simulink model "Force_control_compliance"  (R2020b)
settings: Solver=VariableStepAuto  StartTime=0.0  StopTime=10.0  RelTol=1e-3
settings Model: Creator=Anna Rothweil  LastModifiedBy=Anna Rothweil
settings DebuggingCC: UnderSpecifiedDimensionMsg=warning
settings SFSimCC: CustomCodeUndefinedFunction=UseInterfaceOnly

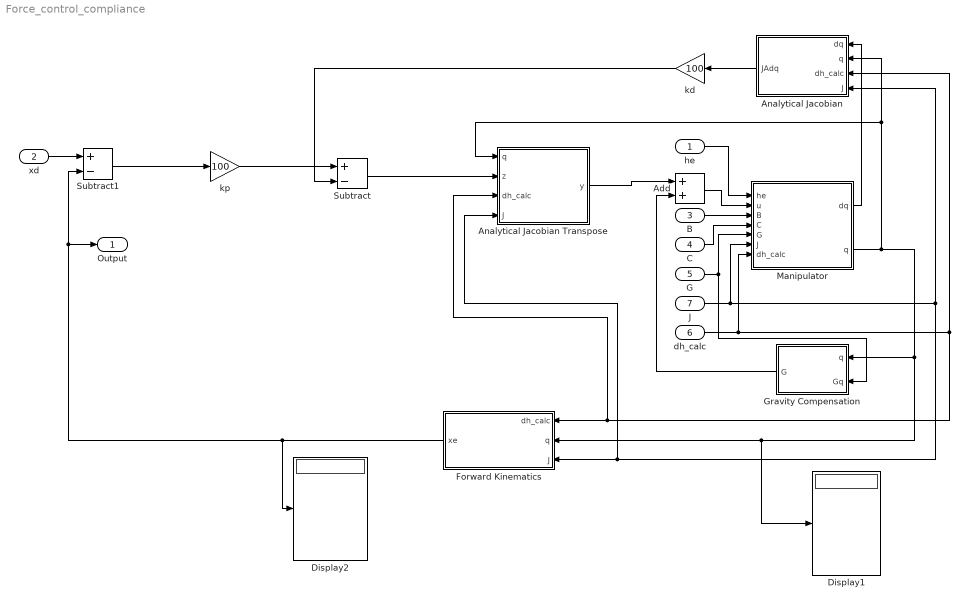
== system Force_control_compliance ==
  he : Inport
  xd : Inport  Port=2
  B : Inport  Port=3
  C : Inport  Port=4
  G : Inport  Port=5
  dh_calc : Inport  Port=6  PortDimensions=12
  J : Inport  Port=7
  Add : Sum
  Analytical Jacobian : MATLAB Function  TreatAsAtomicUnit=on
  "Analytical Jacobian Transpose " : MATLAB Function  TreatAsAtomicUnit=on
  Display1 : Display
  Display2 : Display
  "Forward Kinematics " : MATLAB Function  TreatAsAtomicUnit=on
  "Gravity Compensation " : MATLAB Function  TreatAsAtomicUnit=on
  Manipulator : Subsystem
  Subtract : Sum  Inputs=+-
  Subtract1 : Sum  Inputs=+-
  kd : Gain  Gain=100
  "kp " : Gain  Gain=100
  Output : Outport
  wires:
  Subtract1/1 -> "kp "/1
  "Gravity Compensation "/1(G) -> Add/2
  Subtract/1 -> "Analytical Jacobian Transpose "/2(z)
  "Analytical Jacobian Transpose "/1(y) -> Add/1
  kd/1 -> Subtract/2
  "kp "/1 -> Subtract/1
  xd/1 -> Subtract1/1
  dh_calc/1 -> Manipulator/7(dh_calc), "Analytical Jacobian Transpose "/3(dh_calc), "Forward Kinematics "/1(dh_calc), Analytical Jacobian/3(dh_calc)
  Manipulator/1(dq) -> Analytical Jacobian/1(dq)
  Manipulator/2("q ") -> "Analytical Jacobian Transpose "/1(q), Analytical Jacobian/2(q), Display1/1, "Forward Kinematics "/2(q), "Gravity Compensation "/1(q)
  Add/1 -> Manipulator/2(u)
  he/1 -> Manipulator/1(he)
  "Forward Kinematics "/1(xe) -> Output/1, Subtract1/2, Display2/1
  B/1 -> Manipulator/3(B)
  C/1 -> Manipulator/4(C)
  G/1 -> "Gravity Compensation "/2(Gq), Manipulator/5(G)
  Analytical Jacobian/1(JAdq) -> kd/1
  J/1 -> Manipulator/6(J), "Analytical Jacobian Transpose "/4(J), "Forward Kinematics "/3(J), Analytical Jacobian/4(J)

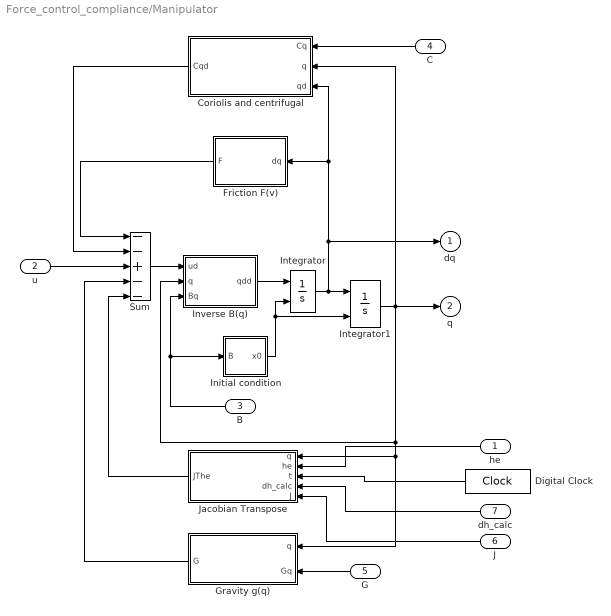
== system Force_control_compliance/Manipulator ==
  he : Inport
  u : Inport  Port=2
  B : Inport  Port=3
  C : Inport  Port=4
  G : Inport  Port=5
  J : Inport  Port=6
  dh_calc : Inport  Port=7
  Coriolis and centrifugal : MATLAB Function  TreatAsAtomicUnit=on
  Digital Clock : DigitalClock  SampleTime=0.001
  Friction F(v) : MATLAB Function  TreatAsAtomicUnit=on
  Gravity g(q) : MATLAB Function  TreatAsAtomicUnit=on
  Initial condition : MATLAB Function  TreatAsAtomicUnit=on
  Integrator : Integrator  InitialConditionSource=external  InitialCondition=[0 0 0 0 0 0]  ZeroCross=off
  Integrator1 : Integrator  InitialConditionSource=external  InitialCondition=[0 0 0 0 0 0]  ZeroCross=off
  Inverse B(q) : MATLAB Function  TreatAsAtomicUnit=on
  Jacobian Transpose : MATLAB Function  TreatAsAtomicUnit=on
  Sum : Sum  Inputs=--+--  InputSameDT=on  SaturateOnIntegerOverflow=on  OutDataTypeStr=Inherit: Same as first input
  dq : Outport  InitialOutput=0
  "q " : Outport  Port=2  InitialOutput=0
  wires:
  Inverse B(q)/1(qdd) -> Integrator/1
  Integrator/1 -> dq/1, Coriolis and centrifugal/3(qd), Friction F(v)/1(dq), Integrator1/1
  Coriolis and centrifugal/1(Cqd) -> Sum/2
  Friction F(v)/1(F) -> Sum/1
  u/1 -> Sum/3
  Integrator1/1 -> Coriolis and centrifugal/2(q), "q "/1, Inverse B(q)/2(q), Gravity g(q)/1(q), Jacobian Transpose/1(q)
  Gravity g(q)/1(G) -> Sum/4
  Jacobian Transpose/1(JThe) -> Sum/5
  he/1 -> Jacobian Transpose/2(he)
  Sum/1 -> Inverse B(q)/1(ud)
  Digital Clock/1 -> Jacobian Transpose/3(t)
  C/1 -> Coriolis and centrifugal/1(Cq)
  B/1 -> Inverse B(q)/3(Bq), Initial condition/1(B)
  G/1 -> Gravity g(q)/2(Gq)
  J/1 -> Jacobian Transpose/5(J)
  dh_calc/1 -> Jacobian Transpose/4(dh_calc)
  Initial condition/1(x0) -> Integrator1/2, Integrator/2

== matlab function Force_control_compliance/Manipulator/Coriolis and centrifugal ==
  data: Cq input; q input; Cqd output; qd input
function Cqd = fcn(Cq, q, qd)
coder.extrinsic('CFinder');
n=size(q, 1);
C = zeros(n,n);
C = CFinder(Cq, q, qd);
Cqd=zeros(n,1);
Cqd=C*qd;

== matlab function Force_control_compliance/Analytical Jacobian Transpose  ==
  data: q input; z input; y output; dh_calc input; J input
function y = fcn(q, z, dh_calc, J)
%dh_calc: the 4*N x 1 vector of symbolic dh parameters (numbers)
%convert dh_calc to matrix form of size Nx4
n=size(q,1);
dh_calc2 = zeros(n,4);
w=1;
for j=1:4
    for i=1:n
        dh_calc2(i,j) = dh_calc(w);
        w=w+1;
    end
end

%z must be 6x1
coder.extrinsic('JAFinder');
JA=zeros(6,n);
JA = JAFinder(dh_calc2, q, J);
y=zeros(n,1);
y=JA.'*z;

== matlab function Force_control_compliance/Forward Kinematics  ==
  data: dh_calc input; q input; xe output; J input
function xe = fcn(dh_calc, q, J)
%dh_calc: the 4*N x 1 vector of symbolic dh parameters (numbers)
%convert dh_calc to matrix form of size Nx4
n=[size(dh_calc,1)]/4;
dh_calc2 = zeros(n,4);
w=1;
for j=1:4
    for i=1:n
        dh_calc2(i,j) = dh_calc(w);
        w=w+1;
    end
end

%q: Nx1 matrix of joint parameters
%T: 4x4 homogeneous transformation matrix

%I think this code is not working because Arm is symbolic
%let's evaluate Arm first before using it with fkine
coder.extrinsic('ArmFinder');
xe=zeros(6,1);
xe = ArmFinder(dh_calc2, q, J);

% s=size(xe,1)
% if s==6
%     xe=xe;
% else
%     xe=zeros(6,1)
%     fprintf('xe is zeros - FWD KIN error')
end

== matlab function Force_control_compliance/Manipulator/Gravity g(q) ==
  data: q input; G output; Gq input
function G = fcn(q, Gq)
coder.extrinsic('GFinder');
n=size(q, 1);
G = zeros(n,1);
G = GFinder(Gq, q);

== matlab function Force_control_compliance/Analytical Jacobian ==
  data: dq input; JAdq output; q input; dh_calc input; J input
function JAdq = fcn(dq, q, dh_calc, J)
%dh_calc: the 4*N x 1 vector of symbolic dh parameters (numbers)
%convert dh_calc to matrix form of size Nx4
n=size(q,1);
dh_calc2 = zeros(n,4);
w=1;
for j=1:4
    for i=1:n
        dh_calc2(i,j) = dh_calc(w);
        w=w+1;
    end
end

coder.extrinsic('JAFinder');
JA=zeros(6,n);
JA = JAFinder(dh_calc2, q, J);
JAdq=zeros(6,1);
JAdq=JA*dq;

== matlab function Force_control_compliance/Gravity Compensation  ==
  data: q input; Gq input; G output
function G = fcn(q, Gq)
n=size(q,1);
coder.extrinsic('GFinder');
G = zeros(n,1);
G = GFinder(Gq, q);

== matlab function Force_control_compliance/Manipulator/Jacobian Transpose ==
  data: q input; JThe output; he input; t input; dh_calc input; J input
function JThe = fcn(q, he, t, dh_calc, J)
%dh_calc: the 4*N x 1 vector of symbolic dh parameters (numbers)
%convert dh_calc to matrix form of size Nx4
n=size(q,1);
dh_calc2 = zeros(n,4);
w=1;
for j=1:4
    for i=1:n
        dh_calc2(i,j) = dh_calc(w);
        w=w+1;
    end
end

coder.extrinsic('JFinder');
J=zeros(6,n);
he_calc=zeros(6,1);
[J, he_calc] = JFinder(dh_calc2, q, J, he, t);

JThe=zeros(n,1);
JThe=(J.')*he_calc;

== matlab function Force_control_compliance/Manipulator/Friction F(v) ==
  data: dq input; F output
function F = fcn(dq)
%friction is  constant; need input from user
n=size(dq,1);
F=zeros(n,1);
%F=0*dq;

== matlab function Force_control_compliance/Manipulator/Initial condition ==
  data: B input; x0 output
function x0 = fcn(B)
n=size(B,1);
x0=zeros(1,n);

== matlab function Force_control_compliance/Manipulator/Inverse B(q) ==
  data: ud input; q input; qdd output; Bq input
function qdd = fcn(ud,q, Bq)
%ud and q must be Nx1
%B (Bq) is NxN
coder.extrinsic('BFinder');
n=size(q, 1);
B = zeros(n,n);
B = BFinder(Bq, q);
%Binv is also NxN
Binv=inv(B);
%qdd must be nx1
qdd=zeros(n,1);
qdd=Binv*ud;
